simulink model "lin_v_ctrl_3d"  (Simulink 7.9)
settings: Solver=ode45  StartTime=0.0  StopTime=tend  FixedStep=params.th  MaxStep=0.01  RelTol=1e-6  AbsTol=1e-3
values from neighbouring files (symbols this model uses):
  Gc_pot = 1*tf([2 1], [1 0])    [ctrl_design.m]    (also in ctrl_design_v2.m = 1*tf([1 1], [1 0]))
  T1_ref = params.Teq(params.op)    [ctrl_design.m]    (also in ctrl_design_v2.m)
settings Model: Creator=puri  LastModifiedBy=Manu
settings CodeAppCC: CustomSymbolStrType=$N$R$M_T
settings GRTTargetCC: CodeReplacementLibrary=None  CPPClassGenCompliant=on

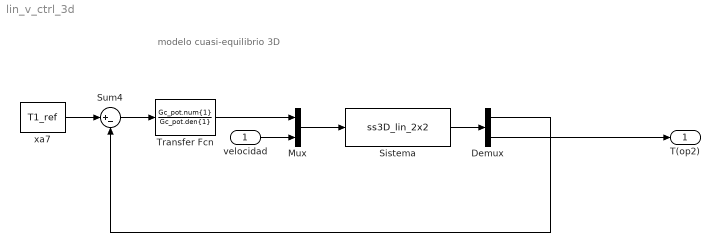
== system lin_v_ctrl_3d ==
  note: modelo cuasi-equilibrio 3D
  velocidad : Inport
  Demux : Demux  Outputs=2
  Mux : Mux  Inputs=2
  Sistema : S-Function  FunctionName=ss3D_lin_2x2  EnableBusSupport=off
      settings: DeleteFcn=shh = get(0,'ShowHiddenHandles');set(0,'ShowHiddenHandles','on');if ~isempty(findobj('type','figure','name','dblcart1 Animation'));close('dblcart1 Animation'); end;set(0,'ShowHiddenHandles',shh);
  Sum4 : Sum  Inputs=|+-
  Transfer Fcn : TransferFcn  Numerator=Gc_pot.num{1}  Denominator=Gc_pot.den{1}
  xa7 : Constant  Value=T1_ref
  T(op2) : Outport
  wires:
  Mux/1 -> Sistema/1
  Transfer Fcn/1 -> Mux/1
  velocidad/1 -> Mux/2
  Sistema/1 -> Demux/1
  Demux/2 -> T(op2)/1
  Demux/1 -> Sum4/2
  Sum4/1 -> Transfer Fcn/1
  xa7/1 -> Sum4/1
